simulink model "CallPhasePlane"  (R2017b)
settings: Solver=FixedStepAuto  StartTime=0.0  StopTime=10.0  FixedStep=0.08  RelTol=1e-3
libraries: MATLAB_Function_lib x9
settings Model: Creator=hbourbou  LastModifiedBy=hbourbou

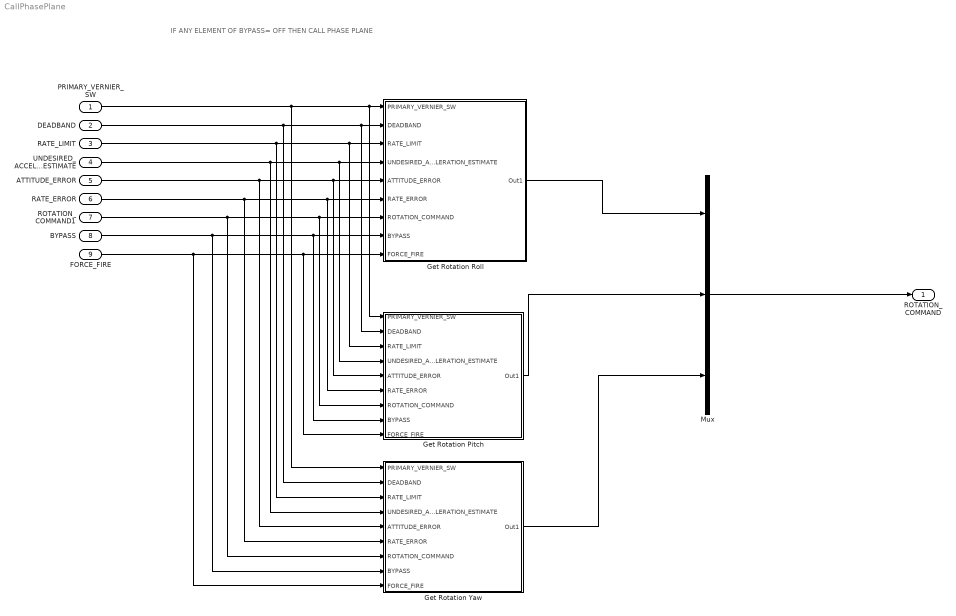
== system CallPhasePlane ==
  note: IF ANY ELEMENT OF BYPASS= OFF THEN CALL PHASE PLANE
  PRIMARY_VERNIER_SW : Inport  OutDataTypeStr=boolean
  DEADBAND : Inport  Port=2
  RATE_LIMIT : Inport  Port=3
  UNDESIRED_ACCELERATION_ESTIMATE : Inport  Port=4
  ATTITUDE_ERROR : Inport  Port=5
  RATE_ERROR : Inport  Port=6
  ROTATION_COMMAND1 : Inport  Port=7
  BYPASS : Inport  Port=8  OutDataTypeStr=boolean  PortDimensions=3
  FORCE_FIRE : Inport  Port=9  OutDataTypeStr=boolean  PortDimensions=3
  Get Rotation Pitch : Subsystem
  Get Rotation Roll : Subsystem
  Get Rotation Yaw : Subsystem
  Mux : Mux  Inputs=3
  ROTATION_COMMAND : Outport
  wires:
  Mux/1 -> ROTATION_COMMAND/1
  Get Rotation Yaw/1(Out1) -> Mux/3
  Get Rotation Pitch/1(Out1) -> Mux/2
  FORCE_FIRE/1 -> Get Rotation Yaw/9(FORCE_FIRE), Get Rotation Pitch/9(FORCE_FIRE), Get Rotation Roll/9(FORCE_FIRE)
  ATTITUDE_ERROR/1 -> Get Rotation Yaw/5(ATTITUDE_ERROR), Get Rotation Pitch/5(ATTITUDE_ERROR), Get Rotation Roll/5(ATTITUDE_ERROR)
  BYPASS/1 -> Get Rotation Yaw/8(BYPASS), Get Rotation Roll/8(BYPASS), Get Rotation Pitch/8(BYPASS)
  PRIMARY_VERNIER_SW/1 -> Get Rotation Yaw/1(PRIMARY_VERNIER_SW), Get Rotation Pitch/1(PRIMARY_VERNIER_SW), Get Rotation Roll/1(PRIMARY_VERNIER_SW)
  UNDESIRED_ACCELERATION_ESTIMATE/1 -> Get Rotation Yaw/4(UNDESIRED_ACCELERATION_ESTIMATE), Get Rotation Roll/4(UNDESIRED_ACCELERATION_ESTIMATE), Get Rotation Pitch/4(UNDESIRED_ACCELERATION_ESTIMATE)
  RATE_ERROR/1 -> Get Rotation Yaw/6(RATE_ERROR), Get Rotation Roll/6(RATE_ERROR), Get Rotation Pitch/6(RATE_ERROR)
  ROTATION_COMMAND1/1 -> Get Rotation Yaw/7(ROTATION_COMMAND), Get Rotation Roll/7(ROTATION_COMMAND), Get Rotation Pitch/7(ROTATION_COMMAND)
  Get Rotation Roll/1(Out1) -> Mux/1
  DEADBAND/1 -> Get Rotation Yaw/2(DEADBAND), Get Rotation Pitch/2(DEADBAND), Get Rotation Roll/2(DEADBAND)
  RATE_LIMIT/1 -> Get Rotation Yaw/3(RATE_LIMIT), Get Rotation Pitch/3(RATE_LIMIT), Get Rotation Roll/3(RATE_LIMIT)

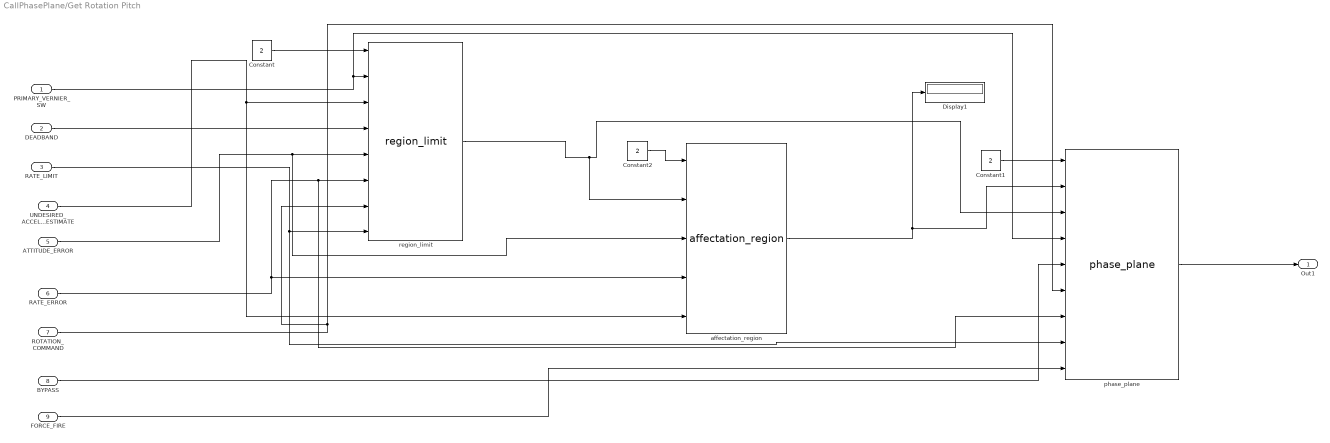
== system CallPhasePlane/Get Rotation Pitch ==
  PRIMARY_VERNIER_SW : Inport
  DEADBAND : Inport  Port=2
  RATE_LIMIT : Inport  Port=3
  UNDESIRED_ACCELERATION_ESTIMATE : Inport  Port=4
  ATTITUDE_ERROR : Inport  Port=5
  RATE_ERROR : Inport  Port=6
  ROTATION_COMMAND : Inport  Port=7
  BYPASS : Inport  Port=8
  FORCE_FIRE : Inport  Port=9
  Constant : Constant  Value=2
  Constant1 : Constant  Value=2
  Constant2 : Constant  Value=2
  Display1 : Display
  affectation_region : MATLAB_Function_lib/affectation_region
  phase_plane : MATLAB_Function_lib/phase_plane
  region_limit : MATLAB_Function_lib/region_limit
  Out1 : Outport
  wires:
  phase_plane/1 -> Out1/1
  Constant/1 -> region_limit/1
  region_limit/1 -> phase_plane/3, affectation_region/2
  BYPASS/1 -> phase_plane/5
  affectation_region/1 -> phase_plane/2, Display1/1
  Constant1/1 -> phase_plane/1
  FORCE_FIRE/1 -> phase_plane/9
  Constant2/1 -> affectation_region/1
  RATE_LIMIT/1 -> phase_plane/8, region_limit/8
  ROTATION_COMMAND/1 -> phase_plane/6, region_limit/7
  RATE_ERROR/1 -> affectation_region/4, phase_plane/7, region_limit/6
  ATTITUDE_ERROR/1 -> affectation_region/3, region_limit/5
  DEADBAND/1 -> region_limit/4
  UNDESIRED_ACCELERATION_ESTIMATE/1 -> affectation_region/5, region_limit/3
  PRIMARY_VERNIER_SW/1 -> phase_plane/4, region_limit/2

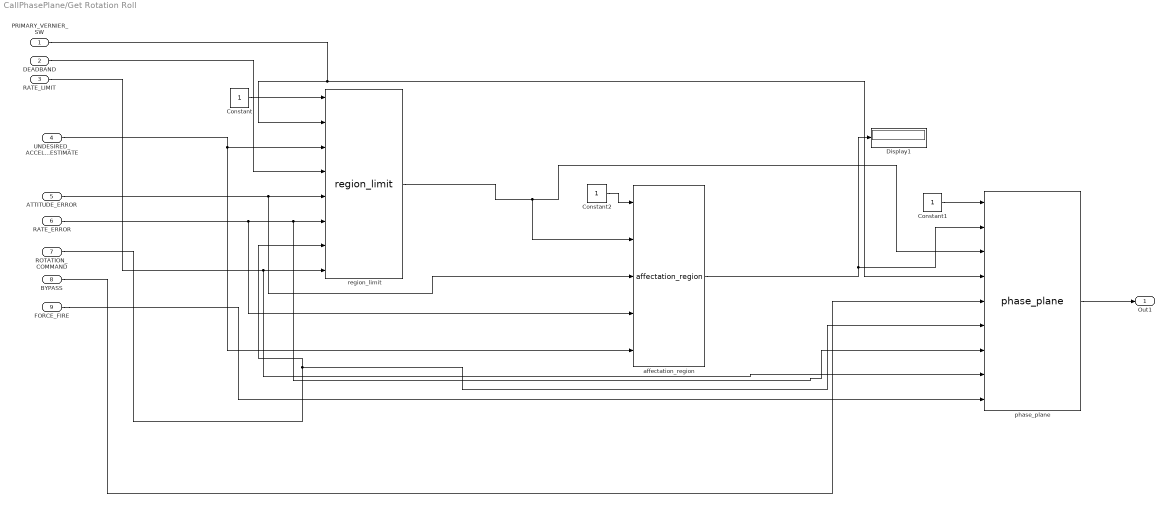
== system CallPhasePlane/Get Rotation Roll ==
  PRIMARY_VERNIER_SW : Inport
  DEADBAND : Inport  Port=2
  RATE_LIMIT : Inport  Port=3
  UNDESIRED_ACCELERATION_ESTIMATE : Inport  Port=4
  ATTITUDE_ERROR : Inport  Port=5
  RATE_ERROR : Inport  Port=6
  ROTATION_COMMAND : Inport  Port=7
  BYPASS : Inport  Port=8
  FORCE_FIRE : Inport  Port=9
  Constant : Constant
  Constant1 : Constant
  Constant2 : Constant
  Display1 : Display
  affectation_region : MATLAB_Function_lib/affectation_region
  phase_plane : MATLAB_Function_lib/phase_plane
  region_limit : MATLAB_Function_lib/region_limit
  Out1 : Outport
  wires:
  phase_plane/1 -> Out1/1
  Constant/1 -> region_limit/1
  region_limit/1 -> phase_plane/3, affectation_region/2
  BYPASS/1 -> phase_plane/5
  affectation_region/1 -> phase_plane/2, Display1/1
  Constant1/1 -> phase_plane/1
  FORCE_FIRE/1 -> phase_plane/9
  Constant2/1 -> affectation_region/1
  RATE_LIMIT/1 -> region_limit/8, phase_plane/8
  ROTATION_COMMAND/1 -> phase_plane/6, region_limit/7
  RATE_ERROR/1 -> affectation_region/4, phase_plane/7, region_limit/6
  ATTITUDE_ERROR/1 -> affectation_region/3, region_limit/5
  DEADBAND/1 -> region_limit/4
  UNDESIRED_ACCELERATION_ESTIMATE/1 -> affectation_region/5, region_limit/3
  PRIMARY_VERNIER_SW/1 -> phase_plane/4, region_limit/2

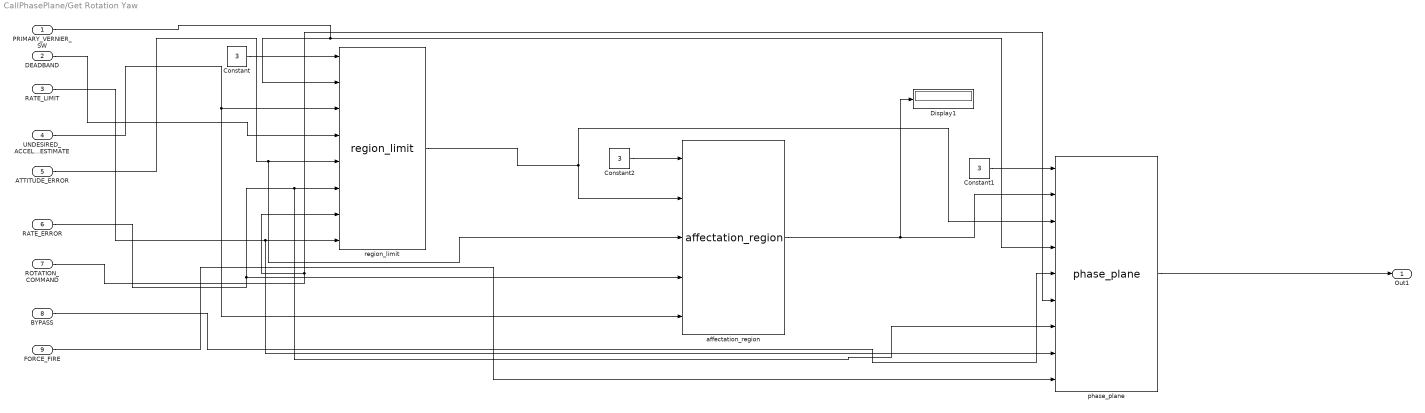
== system CallPhasePlane/Get Rotation Yaw ==
  PRIMARY_VERNIER_SW : Inport
  DEADBAND : Inport  Port=2
  RATE_LIMIT : Inport  Port=3
  UNDESIRED_ACCELERATION_ESTIMATE : Inport  Port=4
  ATTITUDE_ERROR : Inport  Port=5
  RATE_ERROR : Inport  Port=6
  ROTATION_COMMAND : Inport  Port=7
  BYPASS : Inport  Port=8
  FORCE_FIRE : Inport  Port=9
  Constant : Constant  Value=3
  Constant1 : Constant  Value=3
  Constant2 : Constant  Value=3
  Display1 : Display
  affectation_region : MATLAB_Function_lib/affectation_region
  phase_plane : MATLAB_Function_lib/phase_plane
  region_limit : MATLAB_Function_lib/region_limit
  Out1 : Outport
  wires:
  phase_plane/1 -> Out1/1
  Constant/1 -> region_limit/1
  region_limit/1 -> phase_plane/3, affectation_region/2
  BYPASS/1 -> phase_plane/5
  affectation_region/1 -> phase_plane/2, Display1/1
  Constant1/1 -> phase_plane/1
  FORCE_FIRE/1 -> phase_plane/9
  Constant2/1 -> affectation_region/1
  RATE_LIMIT/1 -> phase_plane/8, region_limit/8
  ROTATION_COMMAND/1 -> phase_plane/6, region_limit/7
  RATE_ERROR/1 -> affectation_region/4, phase_plane/7, region_limit/6
  ATTITUDE_ERROR/1 -> affectation_region/3, region_limit/5
  DEADBAND/1 -> region_limit/4
  UNDESIRED_ACCELERATION_ESTIMATE/1 -> affectation_region/5, region_limit/3
  PRIMARY_VERNIER_SW/1 -> phase_plane/4, region_limit/2
